simulink model "Quarter_Car_model"  (R2023b)
settings: Solver=VariableStepAuto  StartTime=0.0  StopTime=10  RelTol=1e-3
model workspace (MAT data in the model file):
  c_s = Simulink.Parameter
  c_s.Value = 237.5
  c_s.Description = 'Shock damping from TG19 Spring Sheet'
  c_s.DataType = 'auto'
  c_s.DocUnits = 'kg/s'
  c_s.Complexity = 'real'
  c_s.Dimensions = [1 1]
  k_s = Simulink.Parameter
  k_s.Value = 3159.177
  k_s.Description = 'Spring stiffness * MR^2 (Wheel Rate (N/m) from TG19 Spring Sheet)'
  k_s.DataType = 'auto'
  k_s.DocUnits = 'N/m'
  k_s.Complexity = 'real'
  k_s.Dimensions = [1 1]
  k_w = Simulink.Parameter
  k_w.Value = 15000
  k_w.Description = 'Tire Spring Stiffness (from internet value)'
  k_w.DataType = 'auto'
  k_w.DocUnits = 'N/m'
  k_w.Complexity = 'real'
  k_w.Dimensions = [1 1]
  m_s = Simulink.Parameter
  m_s.Value = 41
  m_s.Description = 'Sprung corner mass from TG19 Spring Sheet'
  m_s.DataType = 'auto'
  m_s.DocUnits = 'kg'
  m_s.Complexity = 'real'
  m_s.Dimensions = [1 1]
  m_w = Simulink.Parameter
  m_w.Value = 30
  m_w.Description = 'Corner unsprung mass from TG19 Spring Sheet'
  m_w.DataType = 'auto'
  m_w.DocUnits = 'kg'
  m_w.Complexity = 'real'
  m_w.Dimensions = [1 1]
undefined symbols (not defined in the file or in its folder): pulse
libraries: simulink x1
settings Model: Creator=arnav  LastModifiedBy=arnav

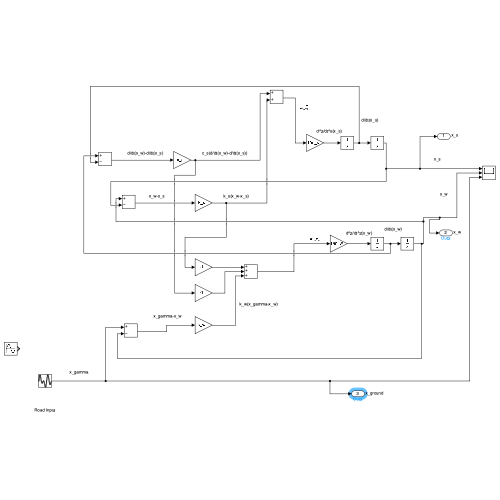
[thumbnail: Simulink's stored preview of the top-level diagram]
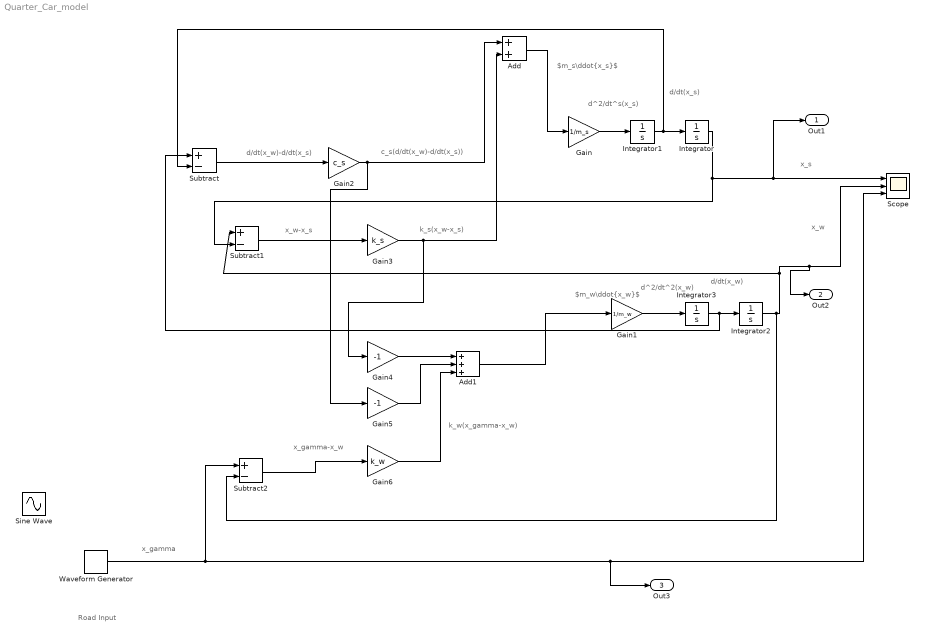
== system Quarter_Car_model ==
  note: x_gamma-x_w
  note: k_w(x_gamma-x_w)
  note: c_s(d/dt(x_w)-d/dt(x_s))
  note: d/dt(x_w)-d/dt(x_s)
  note: $m_s\ddot{x_s}$
  note: d^2/dt^s(x_s)
  note: d/dt(x_w)
  note: x_w
  note: d/dt(x_s)
  note: x_s
  note: x_gamma
  note: Road Input
  note: $m_w\ddot{x_w}$
  note: x_w-x_s
  note: k_s(x_w-x_s)
  note: d^2/dt^2(x_w)
  Add : Sum
  Add1 : Sum  Inputs=+++
  Gain : Gain  Gain=1/m_s
  Gain1 : Gain  Gain=1/m_w
  Gain2 : Gain  Gain=c_s
  Gain3 : Gain  Gain=k_s
  Gain4 : Gain  Gain=-1
  Gain5 : Gain  Gain=-1
  Gain6 : Gain  Gain=k_w
  Integrator{,1..3} (4 alike) : Integrator
  Scope : Scope  NumInputPorts=3
  Sine Wave : Sin  SampleTime=0
  Subtract : Sum  Inputs=+-
  Subtract1 : Sum  Inputs=+-
  Subtract2 : Sum  Inputs=+-
  Waveform Generator : simulink/Sources/Waveform Generator  OutMin=[]  OutMax=[]  OutDataTypeStr=double  SelectedSignal=1  Signals=pulse(0.5,4,0)  BlockNames=MultiportSwitch_462cb53b149d4cf  SampleTime=0.1
  Out1 : Outport  SignalName=x_s
  Out2 : Outport  Port=2  SignalName=x_w
  Out3 : Outport  Port=3  SignalName=x_ground
  wires:
  Waveform Generator/1 -> Subtract2/1, Out3/1, Scope/3
  Integrator/1 -> Out1/1, Scope/1, Subtract1/2
  Integrator3/1 -> Subtract/1, Integrator2/1
  Gain/1 -> Integrator1/1
  Add/1 -> Gain/1
  Gain1/1 -> Integrator3/1
  Integrator1/1 -> Integrator/1, Subtract/2
  Subtract/1 -> Gain2/1
  Gain2/1 -> Gain5/1, Add/1
  Integrator2/1 -> Subtract2/2, Subtract1/1, Out2/1, Scope/2
  Gain3/1 -> Gain4/1, Add/2
  Subtract1/1 -> Gain3/1
  Add1/1 -> Gain1/1
  Gain4/1 -> Add1/1
  Gain5/1 -> Add1/2
  Gain6/1 -> Add1/3
  Subtract2/1 -> Gain6/1
